simulink model "certus_screening"  (R2026a)
settings: Solver=FixedStepDiscrete  StartTime=0  StopTime=p.T_min  FixedStep=p.dt_min
values from neighbouring files (symbols this model uses):
  p = certus_params()    [build_certus_screening.m]    (also in certus_params.m = struct())
settings Model: Creator=nikunj  LastModifiedBy=nikunj

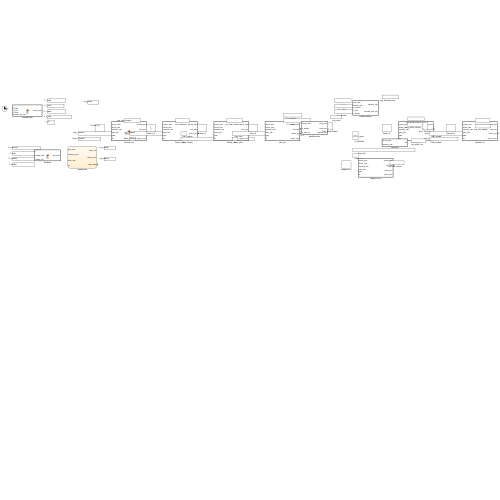
[thumbnail: Simulink's stored preview of the top-level diagram]
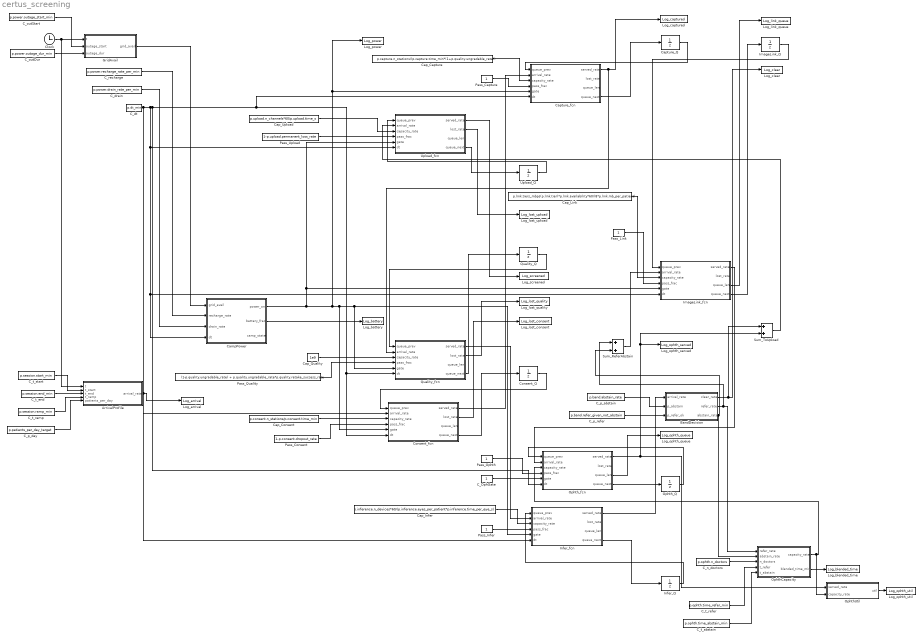
== system certus_screening ==
  ArrivalProfile : MATLAB Function  TreatAsAtomicUnit=on
  BandDecision : MATLAB Function  TreatAsAtomicUnit=on
  C_OphGate : Constant
  C_drain : Constant  Value=p.power.drain_rate_per_min
  C_dt : Constant  Value=p.dt_min
  C_n_doctors : Constant  Value=p.ophth.n_doctors
  C_outDur : Constant  Value=p.power.outage_dur_min
  C_outStart : Constant  Value=p.power.outage_start_min
  C_p_abstain : Constant  Value=p.band.abstain_rate
  C_p_day : Constant  Value=p.patients_per_day_target
  C_p_refer : Constant  Value=p.band.refer_given_not_abstain
  C_recharge : Constant  Value=p.power.recharge_rate_per_min
  C_t_abstain : Constant  Value=p.ophth.time_abstain_min
  C_t_end : Constant  Value=p.session.end_min
  C_t_ramp : Constant  Value=p.session.ramp_min
  C_t_refer : Constant  Value=p.ophth.time_refer_min
  C_t_start : Constant  Value=p.session.start_min
  CampPower : Stateflow chart  TreatAsAtomicUnit=on
  Cap_Capture : Constant  Value=p.capture.n_stations/(p.capture.time_min*(1+p.quality.ungradable_rate))
  Cap_Consent : Constant  Value=p.consent.n_stations/p.consent.time_min
  Cap_Infer : Constant  Value=p.inference.n_devices*60/(p.inference.eyes_per_patient*p.inference.time_per_eye_s)
  Cap_Link : Constant  Value=p.link.tiers_mbps(p.link.tier)*p.link.availability*60/(8*p.link.mb_per_patient)
  Cap_Quality : Constant  Value=1e9
  Cap_Upload : Constant  Value=p.upload.n_channels*60/p.upload.time_s
  Capture_Q : UnitDelay  SampleTime=-1
  Capture_fcn : MATLAB Function  TreatAsAtomicUnit=on
  Clock : Clock
  Consent_Q : UnitDelay  SampleTime=-1
  Consent_fcn : MATLAB Function  TreatAsAtomicUnit=on
  GridAvail : MATLAB Function  TreatAsAtomicUnit=on
  ImageLink_Q : UnitDelay  SampleTime=-1
  ImageLink_fcn : MATLAB Function  TreatAsAtomicUnit=on
  Infer_Q : UnitDelay  SampleTime=-1
  Infer_fcn : MATLAB Function  TreatAsAtomicUnit=on
  Log_arrival : ToWorkspace  VariableName=Log_arrival  SampleTime=p.dt_min
  Log_battery : ToWorkspace  VariableName=Log_battery  SampleTime=p.dt_min
  Log_blended_time : ToWorkspace  VariableName=Log_blended_time  SampleTime=p.dt_min
  Log_captured : ToWorkspace  VariableName=Log_captured  SampleTime=p.dt_min
  Log_clear : ToWorkspace  VariableName=Log_clear  SampleTime=p.dt_min
  Log_link_queue : ToWorkspace  VariableName=Log_link_queue  SampleTime=p.dt_min
  Log_lost_consent : ToWorkspace  VariableName=Log_lost_consent  SampleTime=p.dt_min
  Log_lost_quality : ToWorkspace  VariableName=Log_lost_quality  SampleTime=p.dt_min
  Log_lost_upload : ToWorkspace  VariableName=Log_lost_upload  SampleTime=p.dt_min
  Log_ophth_queue : ToWorkspace  VariableName=Log_ophth_queue  SampleTime=p.dt_min
  Log_ophth_served : ToWorkspace  VariableName=Log_ophth_served  SampleTime=p.dt_min
  Log_ophth_util : ToWorkspace  VariableName=Log_ophth_util  SampleTime=p.dt_min
  Log_power : ToWorkspace  VariableName=Log_power  SampleTime=p.dt_min
  Log_screened : ToWorkspace  VariableName=Log_screened  SampleTime=p.dt_min
  OphthCapacity : MATLAB Function  TreatAsAtomicUnit=on
  OphthUtil : MATLAB Function  TreatAsAtomicUnit=on
  Ophth_Q : UnitDelay  SampleTime=-1
  Ophth_fcn : MATLAB Function  TreatAsAtomicUnit=on
  Pass_Capture : Constant
  Pass_Consent : Constant  Value=1-p.consent.dropout_rate
  Pass_Infer : Constant
  Pass_Link : Constant
  Pass_Ophth : Constant
  Pass_Quality : Constant  Value=(1-p.quality.ungradable_rate) + p.quality.ungradable_rate*p.quality.retake_success_rate
  Pass_Upload : Constant  Value=1-p.upload.permanent_loss_rate
  Quality_Q : UnitDelay  SampleTime=-1
  Quality_fcn : MATLAB Function  TreatAsAtomicUnit=on
  Sum_ReferAbstain : Sum
  Sum_ToUpload : Sum
  Upload_Q : UnitDelay  SampleTime=-1
  Upload_fcn : MATLAB Function  TreatAsAtomicUnit=on
  wires:
  C_recharge/1 -> CampPower/2(recharge_rate)
  C_outStart/1 -> GridAvail/2(outage_start)
  C_p_day/1 -> ArrivalProfile/5(patients_per_day)
  C_drain/1 -> CampPower/3(drain_rate)
  C_outDur/1 -> GridAvail/3(outage_dur)
  Clock/1 -> ArrivalProfile/1(t), GridAvail/1(t)
  C_n_doctors/1 -> OphthCapacity/3(n_doctors)
  C_t_start/1 -> ArrivalProfile/2(t_start)
  C_t_ramp/1 -> ArrivalProfile/4(t_ramp)
  Ophth_Q/1 -> Ophth_fcn/1(queue_prev)
  Ophth_fcn/1(served_rate) -> Sum_ToUpload/2, Log_ophth_served/1, OphthUtil/1(served_rate)
  CampPower/1(power_on) -> Quality_fcn/5(gate), Infer_fcn/5(gate), Consent_fcn/5(gate), Capture_fcn/5(gate), Log_power/1, ImageLink_fcn/5(gate), Upload_fcn/5(gate)
  Pass_Infer/1 -> Infer_fcn/4(pass_frac)
  C_t_end/1 -> ArrivalProfile/3(t_end)
  GridAvail/1(grid_avail) -> CampPower/1(grid_avail)
  C_dt/1 -> ImageLink_fcn/6(dt), CampPower/4(dt), Upload_fcn/6(dt), Consent_fcn/6(dt), Quality_fcn/6(dt), Capture_fcn/6(dt), Ophth_fcn/6(dt), Infer_fcn/6(dt)
  Sum_ToUpload/1 -> Upload_fcn/2(arrival_rate)
  Pass_Upload/1 -> Upload_fcn/4(pass_frac)
  ArrivalProfile/1(arrival_rate) -> Consent_fcn/2(arrival_rate), Log_arrival/1
  Quality_Q/1 -> Quality_fcn/1(queue_prev)
  Cap_Upload/1 -> Upload_fcn/3(capacity_rate)
  CampPower/2(battery_frac) -> Log_battery/1
  Cap_Quality/1 -> Quality_fcn/3(capacity_rate)
  Capture_fcn/4(queue_next) -> Capture_Q/1
  Pass_Quality/1 -> Quality_fcn/4(pass_frac)
  Cap_Consent/1 -> Consent_fcn/3(capacity_rate)
  Pass_Consent/1 -> Consent_fcn/4(pass_frac)
  Cap_Capture/1 -> Capture_fcn/3(capacity_rate)
  Pass_Capture/1 -> Capture_fcn/4(pass_frac)
  Upload_Q/1 -> Upload_fcn/1(queue_prev)
  Upload_fcn/2(lost_rate) -> Log_lost_upload/1
  Upload_fcn/1(served_rate) -> Log_screened/1
  Upload_fcn/4(queue_next) -> Upload_Q/1
  Quality_fcn/1(served_rate) -> Infer_fcn/2(arrival_rate)
  Quality_fcn/2(lost_rate) -> Log_lost_quality/1
  Quality_fcn/4(queue_next) -> Quality_Q/1
  Consent_fcn/1(served_rate) -> Capture_fcn/2(arrival_rate)
  Consent_fcn/2(lost_rate) -> Log_lost_consent/1
  C_p_abstain/1 -> BandDecision/2(p_abstain)
  Consent_fcn/4(queue_next) -> Consent_Q/1
  BandDecision/2(refer_rate) -> Sum_ReferAbstain/1, OphthCapacity/1(refer_rate)
  Pass_Ophth/1 -> Ophth_fcn/4(pass_frac)
  C_OphGate/1 -> Ophth_fcn/5(gate)
  Cap_Infer/1 -> Infer_fcn/3(capacity_rate)
  Capture_Q/1 -> Capture_fcn/1(queue_prev)
  Capture_fcn/1(served_rate) -> Quality_fcn/2(arrival_rate), Log_captured/1
  Cap_Link/1 -> ImageLink_fcn/3(capacity_rate)
  Pass_Link/1 -> ImageLink_fcn/4(pass_frac)
  C_t_abstain/1 -> OphthCapacity/5(t_abstain)
  Sum_ReferAbstain/1 -> ImageLink_fcn/2(arrival_rate)
  Consent_Q/1 -> Consent_fcn/1(queue_prev)
  BandDecision/1(clear_rate) -> Log_clear/1, Sum_ToUpload/1
  ImageLink_fcn/4(queue_next) -> ImageLink_Q/1
  C_p_refer/1 -> BandDecision/3(p_refer_ok)
  Ophth_fcn/3(queue_len) -> Log_ophth_queue/1
  Infer_Q/1 -> Infer_fcn/1(queue_prev)
  Infer_fcn/1(served_rate) -> BandDecision/1(arrival_rate)
  Ophth_fcn/4(queue_next) -> Ophth_Q/1
  Infer_fcn/4(queue_next) -> Infer_Q/1
  ImageLink_Q/1 -> ImageLink_fcn/1(queue_prev)
  ImageLink_fcn/1(served_rate) -> Ophth_fcn/2(arrival_rate)
  ImageLink_fcn/3(queue_len) -> Log_link_queue/1
  BandDecision/3(abstain_rate) -> Sum_ReferAbstain/2, OphthCapacity/2(abstain_rate)
  C_t_refer/1 -> OphthCapacity/4(t_refer)
  OphthCapacity/1(capacity_rate) -> Ophth_fcn/3(capacity_rate), OphthUtil/2(capacity_rate)
  OphthCapacity/2(blended_time_min) -> Log_blended_time/1
  OphthUtil/1(util) -> Log_ophth_util/1

== matlab function certus_screening/Infer_fcn ==
  data: queue_prev input; served_rate output; arrival_rate input; capacity_rate input; pass_frac input; gate input; dt input; lost_rate output; queue_len output; queue_next output
function [served_rate, lost_rate, queue_len, queue_next] = rate_stage(queue_prev, arrival_rate, capacity_rate, pass_frac, gate, dt)
%RATE_STAGE Generic fluid/rate-based queue update for one pipeline
% stage. queue_prev is fed back from a Unit Delay block (this is
% the discrete-time "integrator" state for the stage).
capacity_count = capacity_rate * gate * dt;
arrival_count = arrival_rate * dt;
available = queue_prev + arrival_count;
attempt = min(available, capacity_count);
served_count = attempt * pass_frac;
lost_count = attempt * (1 - pass_frac);
queue_next = available - attempt;
served_rate = served_count / dt;
lost_rate = lost_count / dt;
queue_len = queue_next;

== matlab function certus_screening/BandDecision ==
  data: arrival_rate input; clear_rate output; p_abstain input; p_refer_ok input; refer_rate output; abstain_rate output
function [clear_rate, refer_rate, abstain_rate] = band_decision(arrival_rate, p_abstain, p_refer_ok)
% Screening-band split. p_abstain measured from trust.json
% (screening_band.measured.*.abstain_rate). p_refer_ok is the ASSUMED
% referable-DR share among non-abstained patients (certus_params.m).
abstain_rate = arrival_rate * p_abstain;
ok_rate = arrival_rate * (1 - p_abstain);
refer_rate = ok_rate * p_refer_ok;
clear_rate = ok_rate - refer_rate;

== matlab function certus_screening/OphthCapacity ==
  data: refer_rate input; capacity_rate output; abstain_rate input; n_doctors input; t_refer input; t_abstain input; blended_time_min output
function [capacity_rate, blended_time_min] = ophth_capacity(refer_rate, abstain_rate, n_doctors, t_refer, t_abstain)
% Blended service-time approximation. When arrivals stop at session close,
% total drops to ~0 and the original code jumped to t_abstain (90s), cutting
% clearing capacity by 60% and producing spurious queue build-ups. Instead,
% fall back to t_refer (the faster path) when no new demand is arriving --
% this is conservative for the capacity estimate (faster clearing = fewer
% patients sent home) and honest: the queue at end-of-day is dominated by
% auto-referred eyes, not abstentions.
total = refer_rate + abstain_rate;
if total > 1e-9
    blended_time_min = (refer_rate*t_refer + abstain_rate*t_abstain) / total;
else
    blended_time_min = t_refer;
end
blended_time_min = max(blended_time_min, 1e-6);
capacity_rate = n_doctors / blended_time_min;

== matlab function certus_screening/ImageLink_fcn ==
  data: queue_prev input; served_rate output; arrival_rate input; capacity_rate input; pass_frac input; gate input; dt input; lost_rate output; queue_len output; queue_next output
function [served_rate, lost_rate, queue_len, queue_next] = rate_stage(queue_prev, arrival_rate, capacity_rate, pass_frac, gate, dt)
%RATE_STAGE Generic fluid/rate-based queue update for one pipeline
% stage. queue_prev is fed back from a Unit Delay block (this is
% the discrete-time "integrator" state for the stage).
capacity_count = capacity_rate * gate * dt;
arrival_count = arrival_rate * dt;
available = queue_prev + arrival_count;
attempt = min(available, capacity_count);
served_count = attempt * pass_frac;
lost_count = attempt * (1 - pass_frac);
queue_next = available - attempt;
served_rate = served_count / dt;
lost_rate = lost_count / dt;
queue_len = queue_next;

== matlab function certus_screening/Ophth_fcn ==
  data: queue_prev input; served_rate output; arrival_rate input; capacity_rate input; pass_frac input; gate input; dt input; lost_rate output; queue_len output; queue_next output
function [served_rate, lost_rate, queue_len, queue_next] = rate_stage(queue_prev, arrival_rate, capacity_rate, pass_frac, gate, dt)
%RATE_STAGE Generic fluid/rate-based queue update for one pipeline
% stage. queue_prev is fed back from a Unit Delay block (this is
% the discrete-time "integrator" state for the stage).
capacity_count = capacity_rate * gate * dt;
arrival_count = arrival_rate * dt;
available = queue_prev + arrival_count;
attempt = min(available, capacity_count);
served_count = attempt * pass_frac;
lost_count = attempt * (1 - pass_frac);
queue_next = available - attempt;
served_rate = served_count / dt;
lost_rate = lost_count / dt;
queue_len = queue_next;

== matlab function certus_screening/OphthUtil ==
  data: served_rate input; util output; capacity_rate input
function util = util_calc(served_rate, capacity_rate)
util = served_rate / max(capacity_rate, 1e-9);
util = min(max(util,0),1);

== matlab function certus_screening/Upload_fcn ==
  data: queue_prev input; served_rate output; arrival_rate input; capacity_rate input; pass_frac input; gate input; dt input; lost_rate output; queue_len output; queue_next output
function [served_rate, lost_rate, queue_len, queue_next] = rate_stage(queue_prev, arrival_rate, capacity_rate, pass_frac, gate, dt)
%RATE_STAGE Generic fluid/rate-based queue update for one pipeline
% stage. queue_prev is fed back from a Unit Delay block (this is
% the discrete-time "integrator" state for the stage).
capacity_count = capacity_rate * gate * dt;
arrival_count = arrival_rate * dt;
available = queue_prev + arrival_count;
attempt = min(available, capacity_count);
served_count = attempt * pass_frac;
lost_count = attempt * (1 - pass_frac);
queue_next = available - attempt;
served_rate = served_count / dt;
lost_rate = lost_count / dt;
queue_len = queue_next;

== matlab function certus_screening/GridAvail ==
  data: t input; grid_avail output; outage_start input; outage_dur input
function grid_avail = grid_avail_fn(t, outage_start, outage_dur)
% 1 = grid present, 0 = grid outage. A single outage window per
% scenario is enough to demonstrate the grid->battery->offline
% Stateflow transitions; see run_certus_screening.m for the
% power-outage scenario values.
if t >= outage_start && t < outage_start + outage_dur
    grid_avail = 0;
else
    grid_avail = 1;
end

== matlab function certus_screening/ArrivalProfile ==
  data: t input; arrival_rate output; t_start input; t_end input; t_ramp input; patients_per_day input
function arrival_rate = arrival_profile(t, t_start, t_end, t_ramp, patients_per_day)
% Trapezoid-shaped registration-rate profile (patients/min) that
% integrates to patients_per_day across one camp session. ASSUMPTION:
% patients trickle in/out over t_ramp minutes at open/close rather than
% arriving as a step function.
dur = t_end - t_start;
plateau = max(dur - 2*t_ramp, eps);
peak = patients_per_day / (t_ramp/2 + plateau + t_ramp/2);
if t < t_start || t > t_end
    arrival_rate = 0;
elseif t < t_start + t_ramp
    arrival_rate = peak * (t - t_start) / t_ramp;
elseif t < t_end - t_ramp
    arrival_rate = peak;
else
    arrival_rate = peak * (t_end - t) / t_ramp;
end

== stateflow chart certus_screening/CampPower ==
  state GRID
    entry: power_on=1; camp_state=1;
    during: battery=min(1,battery+recharge_rate*dt); power_on=1; battery_frac=battery;
  state BATTERY
    entry: camp_state=2;
    during: battery=max(0,battery-drain_rate*dt); power_on=1; battery_frac=battery;
  state OFFLINE
    entry: power_on=0; camp_state=3; battery=0;
    during: battery_frac=battery;
  BATTERY -> GRID [order 1] : [grid_avail]
  (default) -> GRID : {battery=1;}
  OFFLINE -> GRID : [grid_avail]
  GRID -> BATTERY : [~grid_avail]
  BATTERY -> OFFLINE [order 2] : [battery<=0]
  data: grid_avail input; recharge_rate input; drain_rate input; dt input; power_on output; battery_frac output; camp_state output; battery local

== matlab function certus_screening/Consent_fcn ==
  data: queue_prev input; served_rate output; arrival_rate input; capacity_rate input; pass_frac input; gate input; dt input; lost_rate output; queue_len output; queue_next output
function [served_rate, lost_rate, queue_len, queue_next] = rate_stage(queue_prev, arrival_rate, capacity_rate, pass_frac, gate, dt)
%RATE_STAGE Generic fluid/rate-based queue update for one pipeline
% stage. queue_prev is fed back from a Unit Delay block (this is
% the discrete-time "integrator" state for the stage).
capacity_count = capacity_rate * gate * dt;
arrival_count = arrival_rate * dt;
available = queue_prev + arrival_count;
attempt = min(available, capacity_count);
served_count = attempt * pass_frac;
lost_count = attempt * (1 - pass_frac);
queue_next = available - attempt;
served_rate = served_count / dt;
lost_rate = lost_count / dt;
queue_len = queue_next;

== matlab function certus_screening/Capture_fcn ==
  data: queue_prev input; served_rate output; arrival_rate input; capacity_rate input; pass_frac input; gate input; dt input; lost_rate output; queue_len output; queue_next output
function [served_rate, lost_rate, queue_len, queue_next] = rate_stage(queue_prev, arrival_rate, capacity_rate, pass_frac, gate, dt)
%RATE_STAGE Generic fluid/rate-based queue update for one pipeline
% stage. queue_prev is fed back from a Unit Delay block (this is
% the discrete-time "integrator" state for the stage).
capacity_count = capacity_rate * gate * dt;
arrival_count = arrival_rate * dt;
available = queue_prev + arrival_count;
attempt = min(available, capacity_count);
served_count = attempt * pass_frac;
lost_count = attempt * (1 - pass_frac);
queue_next = available - attempt;
served_rate = served_count / dt;
lost_rate = lost_count / dt;
queue_len = queue_next;

== matlab function certus_screening/Quality_fcn ==
  data: queue_prev input; served_rate output; arrival_rate input; capacity_rate input; pass_frac input; gate input; dt input; lost_rate output; queue_len output; queue_next output
function [served_rate, lost_rate, queue_len, queue_next] = rate_stage(queue_prev, arrival_rate, capacity_rate, pass_frac, gate, dt)
%RATE_STAGE Generic fluid/rate-based queue update for one pipeline
% stage. queue_prev is fed back from a Unit Delay block (this is
% the discrete-time "integrator" state for the stage).
capacity_count = capacity_rate * gate * dt;
arrival_count = arrival_rate * dt;
available = queue_prev + arrival_count;
attempt = min(available, capacity_count);
served_count = attempt * pass_frac;
lost_count = attempt * (1 - pass_frac);
queue_next = available - attempt;
served_rate = served_count / dt;
lost_rate = lost_count / dt;
queue_len = queue_next;
